simulink model "Lab3_senales_y_sistemas_2020_a"  (R2020a)
settings: Solver=VariableStepAuto  StartTime=0.0  StopTime=0.100  RelTol=1e-3
settings Model: Creator=andy0  LastModifiedBy=andy0
settings DebuggingCC: SFMachineParentedDataDiag=error

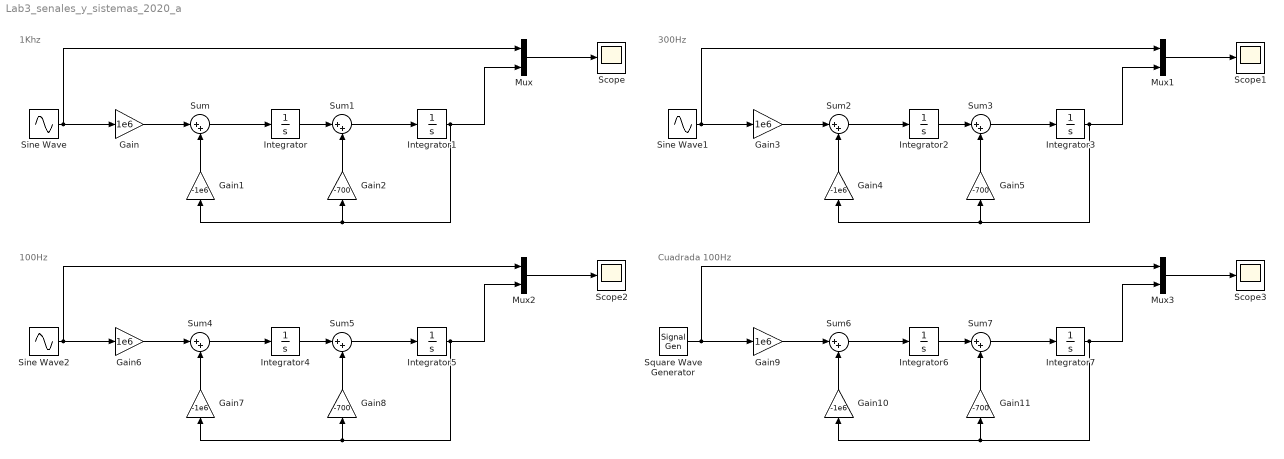
== system Lab3_senales_y_sistemas_2020_a ==
  note: 100Hz
  note: 300Hz
  note: Cuadrada 100Hz
  note: 1Khz
  Gain{,3,6,9} (4 alike) : Gain  Gain=1e6
  Gain{1,4,7,10} (4 alike) : Gain  Gain=-1e6
  Gain{2,5,8,11} (4 alike) : Gain  Gain=-700
  Integrator{,1..7} (8 alike) : Integrator
  Mux{,1..3} (4 alike) : Mux  Inputs=2
  Scope{,1..3} (4 alike) : Scope
  Sine Wave : Sin  Frequency=2*pi*1e3  SampleTime=0.000001
  Sine Wave1 : Sin  Frequency=2*pi*300  SampleTime=0.000001
  Sine Wave2 : Sin  Frequency=2*pi*100  SampleTime=0.000001
  Square Wave Generator : SignalGenerator  WaveForm=square  Frequency=100
  Sum{,1..7} (8 alike) : Sum  Inputs=|++
  wires:
  Mux1/1 -> Scope1/1
  Sine Wave/1 -> Mux/1, Gain/1
  Sum3/1 -> Integrator3/1
  Gain4/1 -> Sum2/2
  Integrator6/1 -> Sum7/1
  Gain10/1 -> Sum6/2
  Gain1/1 -> Sum/2
  Sum2/1 -> Integrator2/1
  Gain/1 -> Sum/1
  Integrator3/1 -> Gain4/1, Gain5/1, Mux1/2
  Mux3/1 -> Scope3/1
  Sum4/1 -> Integrator4/1
  Gain7/1 -> Sum4/2
  Gain5/1 -> Sum3/2
  Sum/1 -> Integrator/1
  Integrator4/1 -> Sum5/1
  Sine Wave1/1 -> Mux1/1, Gain3/1
  Gain2/1 -> Sum1/2
  Integrator2/1 -> Sum3/1
  Sum5/1 -> Integrator5/1
  Integrator5/1 -> Gain7/1, Gain8/1, Mux2/2
  Integrator/1 -> Sum1/1
  Gain9/1 -> Sum6/1
  Sine Wave2/1 -> Mux2/1, Gain6/1
  Gain11/1 -> Sum7/2
  Integrator7/1 -> Gain10/1, Gain11/1, Mux3/2
  Sum6/1 -> Integrator6/1
  Sum7/1 -> Integrator7/1
  Square Wave Generator/1 -> Mux3/1, Gain9/1
  Mux2/1 -> Scope2/1
  Gain6/1 -> Sum4/1
  Gain3/1 -> Sum2/1
  Integrator1/1 -> Gain1/1, Gain2/1, Mux/2
  Gain8/1 -> Sum5/2
  Mux/1 -> Scope/1
  Sum1/1 -> Integrator1/1
